simulink model "MIL_PIL_Simulation_2022"  (R2018b)
settings: Solver=FixedStepAuto  StartTime=0.0  StopTime=5  FixedStep=0.0001  RelTol=1e-3
values from neighbouring files (symbols this model uses):
  F = 1/(C*inv(eye(4)-phi-Gamma*K)*Gamma)    [Controllers.m]    (also in DCMotorController.m = 1/(C_augment*inv(eye(3)-A_augment-B_augment*K)*B_augment); DCRotaryCombined.m = 1/(C_augment*inv(eye(5)-A_augment-B_augment*K)*B_augment); Group_8_assignment1_dc.m = 1/(C_augment*inv(eye(3)-A_augment-B_augment*K)*B_augment); Group_8_assignment1_dual.m = 1/(C_augment*inv(eye(5)-A_augment-B_augment*K)*B_augment))
undefined symbols (not defined in the file or in its folder): A_dp, Ad_plant, B_dp, Bd_plant, C_dp, Cd_plant, D_dp, Dd_plant, delay_count, delay_count_dcmotor, hc, hp, reference, Tp_DC, Ts_DC
libraries: pil_lib x2
settings Model: ExtModeTrigDuration=200  Creator=young  LastModifiedBy=computation
settings DataIOCC: SaveOutput=off  SaveTime=off
settings OptimizationCC: EnhancedBackFolding=on  PassReuseOutputArgsAs=Individual arguments  OptimizeBlockOrder=speed  DifferentSizesBufferReuse=on  OptimizationCustomize=off
settings DebuggingCC: ParameterTunabilityLossMsg=error
settings HardwareCC: ProdBitPerPointer=32  ProdBitPerSizeT=32  ProdBitPerPtrDiffT=32  ProdLargestAtomicInteger=Integer  ProdLargestAtomicFloat=None  ProdWordSize=32  ProdLongLongMode=on  ProdHWDeviceType=Custom Processor
settings SFSimCC: SimUseLocalCustomCode=off  MATLABDynamicMemAlloc=off
settings RTWCC: SystemTargetFile=CompSOC_ec.tlc  TemplateMakefile=CompSOC_ec.tmf  Description=CompSOC EC Target  RTWUseLocalCustomCode=off  IncludeHyperlinkInReport=on  CreateSILPILBlock=PIL  CodeExecutionProfiling=on  CodeProfilingSaveOptions=AllData  CodeProfilingInstrumentation=detailed
settings CodeAppCC: ForceParamTrailComments=on  IgnoreCustomStorageClasses=off  OperatorAnnotations=on  SimulinkDataObjDesc=on  SFDataObjDesc=on  InsertBlockDesc=on
settings STFCustomTargetCC: TargetLibSuffix=.a  TargetLangStandard=C99 (ISO)  MultiwordLength=256  GenerateSampleERTMain=on  CombineOutputUpdateFcns=on  ERTCustomFileBanners=on  SupportNonInlinedSFcns=off  RemoveResetFunc=on  MATLABClassNameForMDSCustomization=Simulink.SoftwareTarget.ERTCustomization  SystemTargetFile=CompSOC_ec.tlc
settings ERTTargetCC: TargetLangStandard=C99 (ISO)  GenerateSampleERTMain=on  ParMdlRefBuildCompliant=off  CompOptLevelCompliant=off  ConcurrentExecutionCompliant=off  SupportContinuousTime=on  ModelStepFunctionPrototypeControlCompliant=off  CPPClassGenCompliant=off  UseToolchainInfoCompliant=off  ExtMode=on  ExtModeStaticAlloc=on  ExtModeStaticAllocSize=30000  ExtModeMexArgs='10.42.0.229' 1 9878  ERTCustomFileTemplate=CompSOC_ec_file_process.tlc

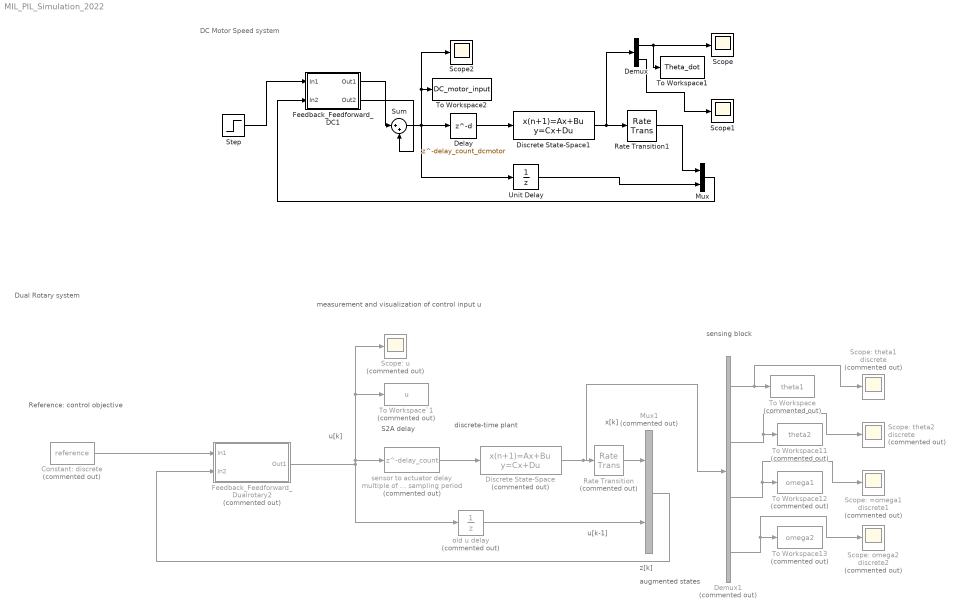
== system MIL_PIL_Simulation_2022 ==
  note: discrete-time plant
  note: sensing block
  note: u[k]
  note: x[k]
  note: measurement and visualization
      | of control input u
  note: augmented states
  note: Reference:
      | control objective
  note: z[k]
  note: u[k-1]
  note: S2A delay
  note: DC Motor Speed system
  note: Dual Rotary system
  Constant: discrete : Constant  Commented=on  Value=reference  OutDataTypeStr=single  SampleTime=hc
  Delay : Delay  DelayLength=delay_count_dcmotor  SampleTime=Tp_DC
  Demux : Demux  Outputs=2
  Demux1 : Demux  Commented=on
  Discrete State-Space : DiscreteStateSpace  Commented=on  A=Ad_plant  B=Bd_plant  C=Cd_plant  D=Dd_plant  SampleTime=hp
  Discrete State-Space1 : DiscreteStateSpace  A=A_dp  B=B_dp  C=C_dp  D=D_dp  SampleTime=Tp_DC
  Feedback_Feedforward_DC1 : Subsystem  DialogController=pil_create_dialog  LoadFcn=|
      | try
      |    if ~strcmp(rtw.pil.getPILVersion, '9.5 (R2018b)_13')
      |       set_param(gcb, 'DialogController', '');
      |       set_param(gcb, 'DialogControllerArgs', '');
      |    end
      | catch e
      |       set_param(gcb, 'DialogController', '');
      |       set_param(gcb, 'DialogControllerArgs', '');
      | end
      mask help: PIL:pil:XILBlockMaskDesc
      mask Display: disp('PIL');
  Feedback_Feedforward_Dualrotary2 : Subsystem  Commented=on
  Mux : Mux  Inputs=2
  Mux1 : Mux  Commented=on  Inputs=2
  Rate Transition : RateTransition  Commented=on  Deterministic=off  OutPortSampleTime=hc
  Rate Transition1 : RateTransition  OutPortSampleTime=Ts_DC
  Scope : Scope
  Scope1 : Scope
  Scope2 : Scope
  Scope: =omega1 discrete1 : Scope  Commented=on
  Scope: omega2 discrete2 : Scope  Commented=on
  Scope: theta1 discrete : Scope  Commented=on
  Scope: theta2 discrete : Scope  Commented=on
  Scope: u : Scope  Commented=on
  Step : Step  Time=0  SampleTime=Ts_DC
  Sum : Sum  Inputs=|++
  To Workspace : ToWorkspace  Commented=on  VariableName=theta1  SaveFormat=Timeseries  SampleTime=hc
  To Workspace1 : ToWorkspace  VariableName=Theta_dot  SaveFormat=Timeseries  SampleTime=Tp_DC
  To Workspace11 : ToWorkspace  Commented=on  VariableName=theta2  SaveFormat=Timeseries  SampleTime=hc
  To Workspace12 : ToWorkspace  Commented=on  VariableName=omega1  SaveFormat=Timeseries  SampleTime=hc
  To Workspace13 : ToWorkspace  Commented=on  VariableName=omega2  SaveFormat=Timeseries  SampleTime=hc
  To Workspace2 : ToWorkspace  VariableName=DC_motor_input  SaveFormat=Timeseries  SampleTime=Ts_DC
  To Workspace`1 : ToWorkspace  Commented=on  VariableName=u  SaveFormat=Timeseries  SampleTime=hc
  Unit Delay : UnitDelay  SampleTime=Ts_DC
  old u delay : UnitDelay  Commented=on  SampleTime=hc
  sensor to actuator delay multiple of plant sampling period : Delay  Commented=on  DelayLength=delay_count  SampleTime=hp
  wires:
  Unit Delay/1 -> Mux/2
  Discrete State-Space/1 -> Rate Transition/1, Demux1/1
  Delay/1 -> Discrete State-Space1/1
  Rate Transition1/1 -> Mux/1
  Sum/1 -> Unit Delay/1, To Workspace2/1, Scope2/1, Delay/1
  Demux1/3 -> Scope: =omega1 discrete1/1, To Workspace12/1
  Rate Transition/1 -> Mux1/1
  old u delay/1 -> Mux1/2
  Demux1/2 -> Scope: theta2 discrete/1, To Workspace11/1
  sensor to actuator delay multiple of plant sampling period/1 -> Discrete State-Space/1
  Demux1/1 -> Scope: theta1 discrete/1, To Workspace/1
  Discrete State-Space1/1 -> Demux/1, Rate Transition1/1
  Demux1/4 -> Scope: omega2 discrete2/1, To Workspace13/1
  Demux/1 -> To Workspace1/1, Scope/1
  Demux/2 -> Scope1/1
  Step/1 -> Feedback_Feedforward_DC1/1(In1)
  Mux/1 -> Feedback_Feedforward_DC1/2(In2)
  Feedback_Feedforward_DC1/1(Out1) -> Sum/1
  Feedback_Feedforward_DC1/2(Out2) -> Sum/2
  Feedback_Feedforward_Dualrotary2/1(Out1) -> sensor to actuator delay multiple of plant sampling period/1, Scope: u/1, To Workspace`1/1, old u delay/1
  Mux1/1 -> Feedback_Feedforward_Dualrotary2/2(In2)
  Constant: discrete/1 -> Feedback_Feedforward_Dualrotary2/1(In1)

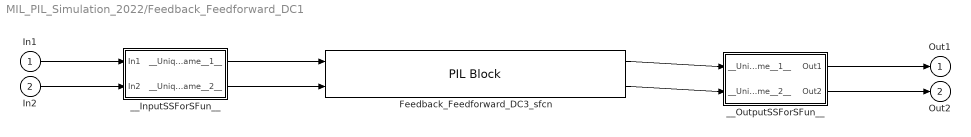
== system MIL_PIL_Simulation_2022/Feedback_Feedforward_DC1 ==
  In1 : Inport
  In2 : Inport  Port=2
  Feedback_Feedforward_DC3_sfcn : pil_lib/PIL Block  SimulationMode=PIL  IsTopModelPIL=off  CodeDir=/media/sf_SharedWork/Feedback_Feedforward_DC3_CompSOC  AnchorDir=/media/sf_SharedWork  ConfigName=CompSOC connectivity config using serial  XrelIsTopModelCode=on  XrelIsReusable=off  XrelDWorkNames={}  XrelDWorkTypes={}  XrelModelArgVals={}  XrelOrderedParamNames={}
  __InputSSForSFun__ : Subsystem
  __OutputSSForSFun__ : Subsystem
  Out1 : Outport
  Out2 : Outport  Port=2
  wires:
  In1/1 -> __InputSSForSFun__/1(In1)
  In2/1 -> __InputSSForSFun__/2(In2)
  __InputSSForSFun__/1(__UniqueOutportName__1__) -> Feedback_Feedforward_DC3_sfcn/1
  __InputSSForSFun__/2(__UniqueOutportName__2__) -> Feedback_Feedforward_DC3_sfcn/2
  Feedback_Feedforward_DC3_sfcn/1 -> __OutputSSForSFun__/1(__UniqueInportName__1__)
  Feedback_Feedforward_DC3_sfcn/2 -> __OutputSSForSFun__/2(__UniqueInportName__2__)
  __OutputSSForSFun__/1(Out1) -> Out1/1
  __OutputSSForSFun__/2(Out2) -> Out2/1

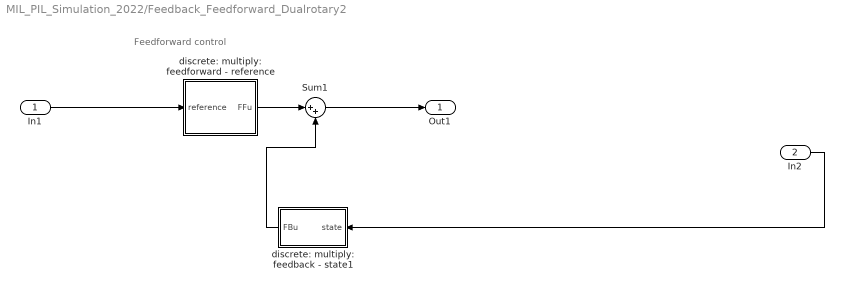
== system MIL_PIL_Simulation_2022/Feedback_Feedforward_Dualrotary2 ==
  note: Feedforward control
  In1 : Inport
  In2 : Inport  Port=2
  Sum1 : Sum  Inputs=|++
  discrete: multiply: feedback - state1 : Subsystem  DialogController=pil_create_dialog  LoadFcn=|
      | try
      |    if ~strcmp(rtw.pil.getPILVersion, '9.5 (R2018b)_13')
      |       set_param(gcb, 'DialogController', '');
      |       set_param(gcb, 'DialogControllerArgs', '');
      |    end
      | catch e
      |       set_param(gcb, 'DialogController', '');
      |       set_param(gcb, 'DialogControllerArgs', '');
      | end
      mask help: PIL:pil:XILBlockMaskDesc
      mask Display: disp('PIL');
  discrete: multiply: feedforward - reference : Subsystem
  Out1 : Outport
  wires:
  In1/1 -> discrete: multiply: feedforward - reference/1(reference)
  discrete: multiply: feedback - state1/1(FBu) -> Sum1/2
  discrete: multiply: feedforward - reference/1(FFu) -> Sum1/1
  Sum1/1 -> Out1/1
  In2/1 -> discrete: multiply: feedback - state1/1(state)

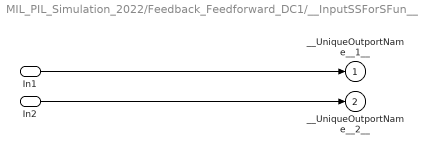
== system MIL_PIL_Simulation_2022/Feedback_Feedforward_DC1/__InputSSForSFun__ ==
  In1 : Inport
  In2 : Inport  Port=2
  __UniqueOutportName__1__ : Outport
  __UniqueOutportName__2__ : Outport  Port=2
  wires:
  In1/1 -> __UniqueOutportName__1__/1
  In2/1 -> __UniqueOutportName__2__/1

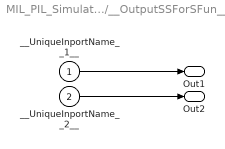
== system MIL_PIL_Simulation_2022/Feedback_Feedforward_DC1/__OutputSSForSFun__ ==
  __UniqueInportName__1__ : Inport
  __UniqueInportName__2__ : Inport  Port=2
  Out1 : Outport
  Out2 : Outport  Port=2
  wires:
  __UniqueInportName__1__/1 -> Out1/1
  __UniqueInportName__2__/1 -> Out2/1

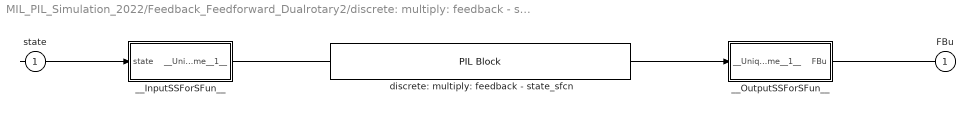
== system MIL_PIL_Simulation_2022/Feedback_Feedforward_Dualrotary2/discrete: multiply: feedback - state1 ==
  state : Inport  OutDataTypeStr=single  SampleTime=hc
  __InputSSForSFun__ : Subsystem
  __OutputSSForSFun__ : Subsystem
  discrete: multiply: feedback - state_sfcn : pil_lib/PIL Block  SimulationMode=PIL  IsTopModelPIL=off  CodeDir=/media/sf_SharedWork/discrete_CompSOC  AnchorDir=/media/sf_SharedWork  ConfigName=CompSOC connectivity config using serial  XrelIsTopModelCode=on  XrelIsReusable=off  XrelDWorkNames={}  XrelDWorkTypes={}  XrelModelArgVals={}  XrelOrderedParamNames={}
  FBu : Outport  OutDataTypeStr=single  SampleTime=hc  InitialOutput=[0]
  wires:
  state/1 -> __InputSSForSFun__/1(state)
  __InputSSForSFun__/1(__UniqueOutportName__1__) -> discrete: multiply: feedback - state_sfcn/1
  discrete: multiply: feedback - state_sfcn/1 -> __OutputSSForSFun__/1(__UniqueInportName__1__)
  __OutputSSForSFun__/1(FBu) -> FBu/1

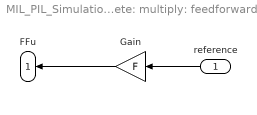
== system MIL_PIL_Simulation_2022/Feedback_Feedforward_Dualrotary2/discrete: multiply: feedforward - reference ==
  reference : Inport  OutDataTypeStr=single  SampleTime=hc
  Gain : Gain  Gain=F  OutDataTypeStr=single
  FFu : Outport  OutDataTypeStr=single  SampleTime=hc  InitialOutput=[0]
  wires:
  reference/1 -> Gain/1
  Gain/1 -> FFu/1

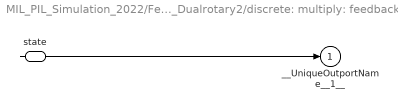
== system MIL_PIL_Simulation_2022/Feedback_Feedforward_Dualrotary2/discrete: multiply: feedback - state1/__InputSSForSFun__ ==
  state : Inport  OutDataTypeStr=single  SampleTime=hc
  __UniqueOutportName__1__ : Outport
  wires:
  state/1 -> __UniqueOutportName__1__/1

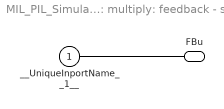
== system MIL_PIL_Simulation_2022/Feedback_Feedforward_Dualrotary2/discrete: multiply: feedback - state1/__OutputSSForSFun__ ==
  __UniqueInportName__1__ : Inport
  FBu : Outport  OutDataTypeStr=single  SampleTime=hc  InitialOutput=[0]
  wires:
  __UniqueInportName__1__/1 -> FBu/1
